simulink model "DCV_tester"  (R2024b)
settings: Solver=FixedStepAuto  StartTime=0.0  StopTime=2  FixedStep=0.01  RelTol=1e-3
libraries: SimscapeFluids_lib x2
settings Model: Creator=Emil  LastModifiedBy=krist

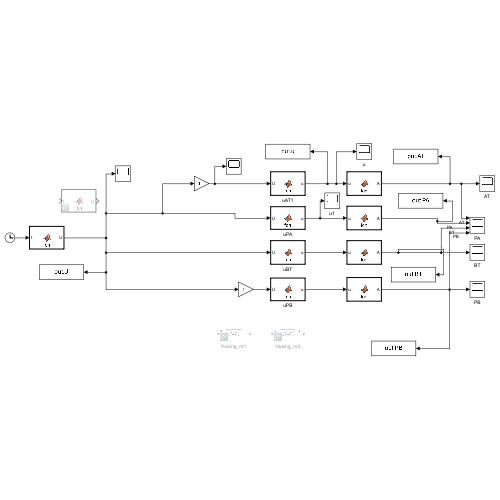
[thumbnail: Simulink's stored preview of the top-level diagram]
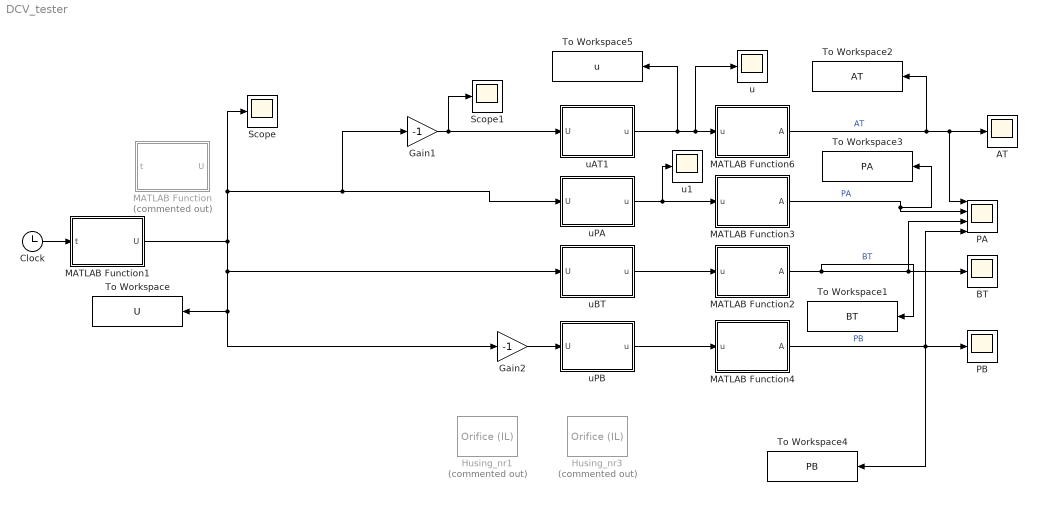
== system DCV_tester ==
  AT : Scope
  BT : Scope
  Clock : Clock
  Gain1 : Gain  Gain=-1
  Gain2 : Gain  Gain=-1
  Husing_nr1 : SimscapeFluids_lib/Isothermal Liquid/Valves & Orifices/Orifices/Orifice (IL)  Commented=on  orifice_type=foundation.enum.constant_variable.constant  constant_orifice_spec=fluids.isothermal_liquid.valves_orifices.orifices.enum.constant_orifice_spec.table1D_volflow_pressure  variable_orifice_spec=fluids.isothermal_liquid.valves_orifices.orifices.enum.orifice_spec.linear  orifice_area_constant=1e-3 m^2  p_diff_TLU_constant=[0, 6/22*5 , 17/22*5, 35/44*10, 60/66*15] bar  vol_flow_TLU_constant="[0, 20, 40, 60, 80]  lpm"  S_min=0 m  del_S=5e-3 m  open_orientation=fluids.isothermal_liquid.valves_orifices.orifices.enum.orifice_orientation.positive  area_max=1e-4 m^2  area_leak=1e-10 m^2  S_TLU=[0, .002, .004, .007, .017] m  orifice_area_TLU=[1e-09, 2.0352e-07, 4.0736e-05, .00011438, .00034356] m^2  area=inf m^2  Cd=0.64  Re_c=150  smoothing_factor=0.01  pressure_recovery=false  S_vol_flow_TLU=[0, .002, .004, .007, .017] m  p_diff_TLU=[.3, .5, .7] MPa  vol_flow_TLU=1e-3 * [1.7e-05, 2e-05, 2.6e-05; .0035, .0045, .0053; .7, .9, 1.06; 1.96, 2.5, 3; 6, 7.7, 9.13] m^3/s
      settings: InternalSimscapePortConfiguration="{\"Bottom\":[],\"Left\":[{\"id\":\"A\",\"label\":\"A\",\"type\":\"foundation.isothermal_liquid.isothermal_liquid\"}],\"Right\":[{\"id\":\"B\",\"label\":\"B\",\"type\":\"foundation.isothermal_liquid.isothermal_liquid\"}],\"Top\":[]}"
  Husing_nr3 : SimscapeFluids_lib/Isothermal Liquid/Valves & Orifices/Orifices/Orifice (IL)  Commented=on  orifice_type=foundation.enum.constant_variable.constant  constant_orifice_spec=fluids.isothermal_liquid.valves_orifices.orifices.enum.constant_orifice_spec.table1D_volflow_pressure  variable_orifice_spec=fluids.isothermal_liquid.valves_orifices.orifices.enum.orifice_spec.linear  orifice_area_constant=1e-3 m^2  p_diff_TLU_constant=[0, 2/22*5 , 7/22*5, 14/22*5, 5, 33/44*10] bar  vol_flow_TLU_constant="[0, 20, 40, 60, 80, 100]  lpm"  S_min=0 m  del_S=5e-3 m  open_orientation=fluids.isothermal_liquid.valves_orifices.orifices.enum.orifice_orientation.positive  area_max=1e-4 m^2  area_leak=1e-10 m^2  S_TLU=[0, .002, .004, .007, .017] m  orifice_area_TLU=[1e-09, 2.0352e-07, 4.0736e-05, .00011438, .00034356] m^2  area=inf m^2  Cd=0.64  Re_c=150  smoothing_factor=0.01  pressure_recovery=false  S_vol_flow_TLU=[0, .002, .004, .007, .017] m  p_diff_TLU=[.3, .5, .7] MPa  vol_flow_TLU=1e-3 * [1.7e-05, 2e-05, 2.6e-05; .0035, .0045, .0053; .7, .9, 1.06; 1.96, 2.5, 3; 6, 7.7, 9.13] m^3/s
      settings: InternalSimscapePortConfiguration="{\"Bottom\":[],\"Left\":[{\"id\":\"A\",\"label\":\"A\",\"type\":\"foundation.isothermal_liquid.isothermal_liquid\"}],\"Right\":[{\"id\":\"B\",\"label\":\"B\",\"type\":\"foundation.isothermal_liquid.isothermal_liquid\"}],\"Top\":[]}"
  MATLAB Function : MATLAB Function  Commented=on  TreatAsAtomicUnit=on
  MATLAB Function1 : MATLAB Function  TreatAsAtomicUnit=on
  MATLAB Function2 : MATLAB Function  TreatAsAtomicUnit=on
  MATLAB Function3 : MATLAB Function  TreatAsAtomicUnit=on
  MATLAB Function4 : MATLAB Function  TreatAsAtomicUnit=on
  MATLAB Function6 : MATLAB Function  TreatAsAtomicUnit=on
  PA : Scope  NumInputPorts=4
  PB : Scope
  Scope : Scope
  Scope1 : Scope
  To Workspace : ToWorkspace  VariableName=U  SampleTime=-1
      settings: Save2DSignal=2-D array (concatenate along first dimension)
  To Workspace1 : ToWorkspace  VariableName=BT  SampleTime=-1
      settings: Save2DSignal=2-D array (concatenate along first dimension)
  To Workspace2 : ToWorkspace  VariableName=AT  SampleTime=-1
      settings: Save2DSignal=2-D array (concatenate along first dimension)
  To Workspace3 : ToWorkspace  VariableName=PA  SampleTime=-1
      settings: Save2DSignal=2-D array (concatenate along first dimension)
  To Workspace4 : ToWorkspace  VariableName=PB  SampleTime=-1
      settings: Save2DSignal=2-D array (concatenate along first dimension)
  To Workspace5 : ToWorkspace  VariableName=u  SampleTime=-1
      settings: Save2DSignal=2-D array (concatenate along first dimension)
  u : Scope
  u1 : Scope
  uAT1 : MATLAB Function  TreatAsAtomicUnit=on
  uBT : MATLAB Function  TreatAsAtomicUnit=on
  uPA : MATLAB Function  TreatAsAtomicUnit=on
  uPB : MATLAB Function  TreatAsAtomicUnit=on
  wires:
  Clock/1 -> MATLAB Function1/1(t)
  Gain2/1 -> uPB/1(U)
  uPA/1(u) -> u1/1, MATLAB Function3/1(u)
  uAT1/1(u) -> To Workspace5/1, MATLAB Function6/1(u), u/1
  uBT/1(u) -> MATLAB Function2/1(u)
  MATLAB Function6/1(A) -> To Workspace2/1, PA/1, AT/1  "AT"
  MATLAB Function2/1(A) -> To Workspace1/1, PA/3, BT/1  "BT"
  MATLAB Function3/1(A) -> PA/2, To Workspace3/1  "PA"
  MATLAB Function4/1(A) -> PA/4, To Workspace4/1, PB/1  "PB"
  uPB/1(u) -> MATLAB Function4/1(u)
  MATLAB Function1/1(U) -> uBT/1(U), Gain2/1, To Workspace/1, Scope/1, Gain1/1, uPA/1(U)
  Gain1/1 -> uAT1/1(U), Scope1/1

== matlab function DCV_tester/MATLAB Function ==
  data: t input; U output
function U = fcn(t)
t_ramp = 1;
t_hold = 0.5;

if t < t_hold
    U = 0;
elseif t < t_ramp+t_hold
    U=1*(t-t_hold)/t_ramp;
elseif t < t_ramp+t_hold*2
    U=1;
elseif t < t_ramp*2+t_hold*2
    U=1-1*(t-t_ramp-t_hold*2)/t_ramp;
elseif t < t_ramp*2+t_hold*3
    U=0;
elseif t < t_ramp*3+t_hold*3
    U=-1*(t-t_ramp*2-t_hold*3)/t_ramp;
elseif t < t_ramp*3+t_hold*4
    U = -1;
elseif t < t_ramp*4+t_hold*4
    U=-1+1*(t-t_ramp*3-t_hold*4)/t_ramp;
else
    U = 0;
end

== matlab function DCV_tester/uPB ==
  data: U input; u output
function u = fcn(U)
if U < 0.15
    u = 0;
elseif U >=0.15
    u= (U-0.15)/(1-0.15);
else
    u = 0;
end

== matlab function DCV_tester/uPA ==
  data: U input; u output
function u = fcn(U)
if U < 0.15
    u = 0;
elseif U >=0.15
    u= (U-0.15)/(1-0.15);
else
    u = 0;
end

== matlab function DCV_tester/uBT ==
  data: U input; u output
function u = fcn(U)
if U < -0.15
    u=0;
elseif U <= 0
    u = 0.15-abs(U);
elseif U < 0.15
    u = 0.15;
elseif U >=0.15
    u= U;
else
    u = 0;
end

== matlab function DCV_tester/MATLAB Function6 ==
  data: u input; A output
function A = fcn(u)
Q_rat = 16/6e4;
dP = 1e5;
cd = 0.64;
rho = 850;
A_0 = Q_rat*0/(cd*sqrt(2/rho*dP));
A_15 = Q_rat*0.15/(cd*sqrt(2/rho*dP));
A_100 = Q_rat*1/(cd*sqrt(2/rho*dP));
% if u < 0
%     A = A_0*1e6;
% elseif 0 < u <0.15
%     A = A_15*u/0.15*1e6;
% elseif u == 0.15
%     A = A_15*1e6;
% elseif u<=1.15
%     A = A_100*1e6 * (u)/1.15;
% else
%     A =0
% end
if u <= 0
    A = 0;
elseif u < 0.15
    U = u-0;
    A  = Q_rat/(cd*sqrt(2/rho*dP))*1e6*U;
elseif u == 0.15
    U = 0.15;
    A  = Q_rat*U/(cd*sqrt(2/rho*dP))*1e6;
elseif u <= 1.15
    U = u;
    A  = (Q_rat/(cd*sqrt(2/rho*dP))-Q_rat*0.15/(cd*sqrt(2/rho*dP)))*1e6*(U-0.15)+Q_rat*0.15/(cd*sqrt(2/rho*dP))*1e6;
else
    A = 0;
end

== matlab function DCV_tester/MATLAB Function2 ==
  data: u input; A output
function A = fcn(u)
Q_rat = 20/6e4;
dP = 1e5;
cd = 0.64;
rho = 850;
A = Q_rat*u/(cd*sqrt(2/rho*dP));
A = A*1e6;

== matlab function DCV_tester/MATLAB Function3 ==
  data: u input; A output
function A = fcn(u)
Q_rat = 20/6e4;
dP = 6e5;
cd = 0.64;
rho = 850;
A = Q_rat*u/(cd*sqrt(2/rho*dP));
A = A*1e6;

== matlab function DCV_tester/MATLAB Function4 ==
  data: u input; A output
function A = fcn(u)
Q_rat = 16/6e4;
dP = 6e5;
cd = 0.64;
rho = 850;
A = Q_rat*u/(cd*sqrt(2/rho*dP));
A = A*1e6;

== matlab function DCV_tester/uAT1 ==
  data: U input; u output
function u = fcn(U)
if U < -0.15
    u=0;
elseif U <= 0
    u = 0.15-abs(U);
elseif U <= 0.15
    u = 0.15;
elseif U >0.15
    u= (U-0.15)/(1-0.15)+0.15;
else
    u = 0;
end
% u = u+0.15;

% function u = fcn(U)
% if U < -0.15
%     u=0;
% elseif U <= 0
%     u = 0.15-abs(U);
% elseif U < 0.15
%     u = 0.15;
% elseif U >=0.15
%     u= U;
% else
%     u = 0;
% end

== matlab function DCV_tester/MATLAB Function1 ==
  data: t input; U output
function U = fcn(t)
U=1-t;
% t_ramp = 0.85;
% t_hold = 0.15;
% 
% if t < t_ramp
%    U = -1 + 1*t/t_ramp;
% elseif t < t_ramp+t_hold*2
%     U  = 0;
% elseif t < t_ramp*2+t_hold*2+1
%     U = 1*(t-t_ramp-t_hold*2)/t_ramp;
% else 
%     U = 1;
% end
%
